simulink model "Eg8_5"  (R2018a)
settings: Solver=VariableStepAuto  StartTime=0.0  StopTime=500  RelTol=1e-3
settings Model: Creator=wangluo  LastModifiedBy=wangluo

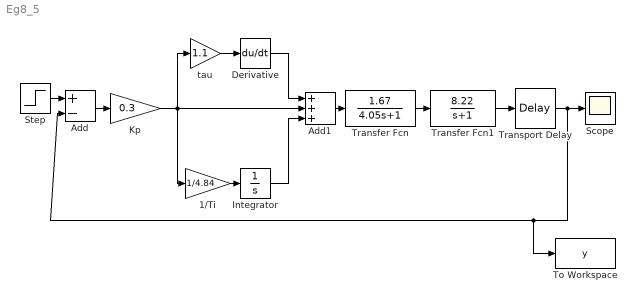
== system Eg8_5 ==
  1/Ti : Gain  Gain=1/4.84
  Add : Sum  Inputs=+-
  Add1 : Sum  Inputs=+++
  Derivative : Derivative
  Integrator : Integrator
  Kp : Gain  Gain=0.3
  Scope : Scope
  Step : Step  SampleTime=0
  To Workspace : ToWorkspace  VariableName=y  SaveFormat=Timeseries  SampleTime=-1
  Transfer Fcn : TransferFcn  Numerator=[1.67]  Denominator=[4.05 1]
  Transfer Fcn1 : TransferFcn  Numerator=[8.22]  Denominator=[1 1]
  Transport Delay : TransportDelay  DelayTime=2.2
  tau : Gain  Gain=1.1
  wires:
  Step/1 -> Add/1
  Add/1 -> Kp/1
  tau/1 -> Derivative/1
  1/Ti/1 -> Integrator/1
  Kp/1 -> tau/1, 1/Ti/1, Add1/2
  Add1/1 -> Transfer Fcn/1
  Transport Delay/1 -> Scope/1, To Workspace/1, Add/2
  Derivative/1 -> Add1/1
  Integrator/1 -> Add1/3
  Transfer Fcn/1 -> Transfer Fcn1/1
  Transfer Fcn1/1 -> Transport Delay/1
